simulink library "PTC_MBDS_ForceMarker"  (R2013a)
settings: Solver=ode1  StartTime=0.0  StopTime=Inf  FixedStep=0.001  RelTol=1e-3
undefined symbols (not defined in the file or in its folder): FeedThrough, PTC_MBDS_GlobalFeedThrough_Fcn, Value
libraries: PTC_MBDS_ForceMarker x1
settings Model: Creator=sundeep.tuteja  LastModifiedBy=Sundeep.Tuteja

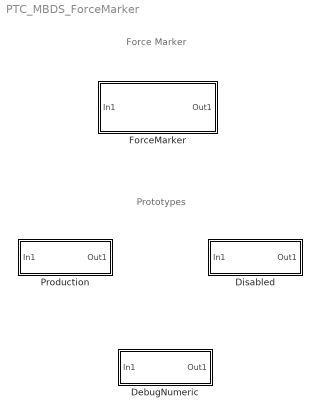
== system PTC_MBDS_ForceMarker ==
  note: Force Marker
  note: Prototypes
  DebugNumeric : Subsystem  BlockChoice=DebugNumeric
  Disabled : Subsystem
  ForceMarker : Subsystem  BlockChoice=DebugNumeric  mask(ForceMarker){MarkerName=, Value=0, FeedThrough=on, Disable=off, PTC_MBDS_BlockVersion=5.31, PTC_BlockType=PTC_MBDS_ForceMarker}
      mask prompts: MarkerName "Name"; FeedThrough "Feed Through"
      mask help: This block implements the Force-Marker according to IEC61131-3.
      mask init:
      | ptc_matlab_lib.PTC_MBDS_BlockCallback('action', 'init');
      settings: AttributesFormatString=FM_%<MarkerName>  CopyFcn=ptc_matlab_lib.PTC_MBDS_BlockCallback('action', 'CopyFcn');  DeleteFcn=ptc_matlab_lib.PTC_MBDS_BlockCallback('action', 'DeleteFcn');  UndoDeleteFcn=ptc_matlab_lib.PTC_MBDS_BlockCallback('action', 'UndoDeleteFcn');  TemplateBlock=self  MemberBlocks=DebugNumeric,Disabled,Production
      mask Help: web(fullfile(fileparts(which('PTC_MBDS_LIB')), 'Help', [get(gcbh, 'PTC_BlockType') '.html']));
      mask Callback MarkerName: ptc_matlab_lib.PTC_MBDS_BlockCallback('ParamVariable', 'MarkerName');
      mask Callback Disable: ptc_matlab_lib.PTC_MBDS_BlockCallback('ParamVariable', 'Disable');
      mask Callback PTC_MBDS_BlockVersion: set(gcbh, 'PTC_MBDS_BlockVersion', PTC_MBDS_Version_Fcn);
      mask TypeOptions PTC_BlockType: PTC_MBDS_ForceMarker
      mask Display:
      | thisPosition = get(gcbh, 'Position');
      | drawDisable = PTC_MBDS_GlobalDisable_Fcn || ...
      |    (Disable && ~PTC_MBDS_GlobalFeedThrough_Fcn);
      | drawFeedThrough = drawDisable || ...
      |    PTC_MBDS_GlobalFeedThrough_Fcn || ...
      |    FeedThrough;
      | drawGlobal = PTC_MBDS_GlobalDisable_Fcn || ...
      |    PTC_MBDS_GlobalFeedThrough_Fcn;
      | drawForceValue = ~drawDisable && ~drawFeedThrough;
      | 
      | if drawFeedThrough
      |    plot(thisPosition([1 3]), mean(thisPosition([2 4])) * ones(1, 2));
      | end
      | 
      | if drawDisable
      |    set(gcbh, 'MaskIconFrame', 'off')
      |    GAP = 15;
      |    DASHLENGTH = 25;
      | 
      |    %Plot top line
      |    startx = thisPosition(1);
      |    endx = startx + DASHLENGTH;
      |    endx = min(endx, thisPosition(3));
      |    while startx <= endx
      |       plot([startx, endx], [thisPosition(4), thisPosition(4)]);
      |       startx = endx + GAP;
      |       endx = startx + DASHLENGTH;
      |       endx = min(endx, thisPosition(3));
      |    end
      | 
      |    %Plot bottom line
      |    startx = thisPosition(1);
      |    endx = startx + DASHLENGTH;
      |    endx = min(endx, thisPosition(3));
      |    while startx <= endx
      |       plot([startx, endx], [thisPosition(2), thisPosition(2)]);
      |       startx = endx + GAP;
      |       endx = startx + DASHLENGTH;
      |       endx = min(endx, thisPosition(3));
      |    end
      | 
      |    %Plot left line
      |    starty = thisPosition(2);
      |    endy = starty + DASHLENGTH;
      |    endy = min(endy, thisPosition(4));
      |    while starty <= endy
      |       plot([thisPosition(1), thisPosition(1)], [starty, endy]);
      |       starty = endy + GAP;
      |       endy = endy + DASHLENGTH;
      |       endy = min(endy, thisPosition(4));
      |    end
      | 
      |    %Plot left line
      |    starty = thisPosition(2);
      |    endy = starty + DASHLENGTH;
      |    endy = min(endy, thisPosition(4));
      |    while starty <= endy
      |       plot([thisPosition(3), thisPosition(3)], [starty, endy]);
      |       starty = endy + GAP;
      |       endy = endy + DASHLENGTH;
      |       endy = min(endy, thisPosition(4));
      |    end
      | end
      | 
      | if ~drawDisable
      |    set(gcbh, 'MaskIconFrame', 'on');
      | end
      | 
      | if drawGlobal
      |    text(mean(thisPosition([1 3])), mean(thisPosition([2 4])), 'global', 'horizontalAlignment', 'center', 'verticalAlignment', 'bottom');
      | end
      | 
      | if drawForceValue
      |    disp(Value);
      | end
  Production : Subsystem

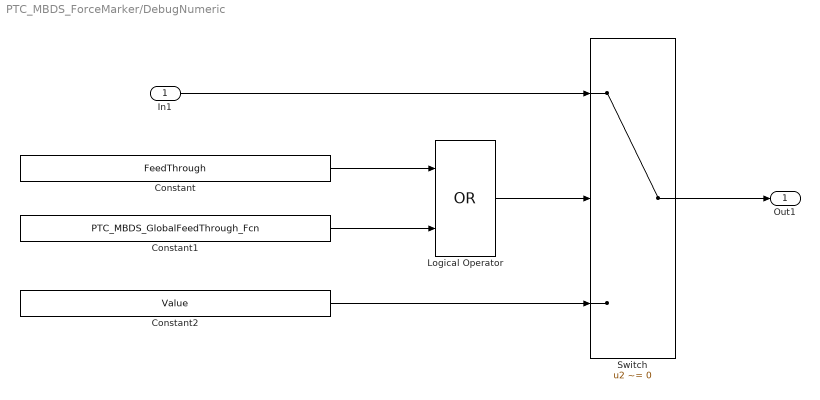
== system PTC_MBDS_ForceMarker/DebugNumeric ==
  In1 : Inport
  Constant : Constant  Value=FeedThrough  OutDataTypeStr=boolean
  Constant1 : Constant  Value=PTC_MBDS_GlobalFeedThrough_Fcn  OutDataTypeStr=boolean
  Constant2 : Constant  Value=Value  OutDataTypeStr=Inherit: Inherit via back propagation
  Logical Operator : Logic  Operator=OR  AllPortsSameDT=off  OutDataTypeStr=boolean
  Switch : Switch  Criteria=u2 ~= 0
  Out1 : Outport
  wires:
  Constant/1 -> Logical Operator/1
  Constant1/1 -> Logical Operator/2
  Constant2/1 -> Switch/3
  Logical Operator/1 -> Switch/2
  Switch/1 -> Out1/1
  In1/1 -> Switch/1

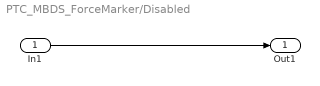
== system PTC_MBDS_ForceMarker/Disabled ==
  In1 : Inport
  Out1 : Outport
  wires:
  In1/1 -> Out1/1

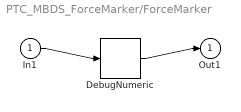
== system PTC_MBDS_ForceMarker/ForceMarker ==
  In1 : Inport
  DebugNumeric : PTC_MBDS_ForceMarker/DebugNumeric
  Out1 : Outport
  wires:
  In1/1 -> DebugNumeric/1
  DebugNumeric/1 -> Out1/1

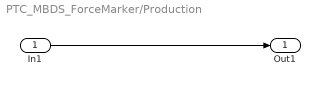
== system PTC_MBDS_ForceMarker/Production ==
  In1 : Inport
  Out1 : Outport
  wires:
  In1/1 -> Out1/1
